simulink model "nona_13_12_simscape_4QC_real"  (R2021b)
settings: Solver=VariableStepAuto  StartTime=0.0  StopTime=10.0  MaxStep=1e-5  RelTol=1e-3
values from neighbouring files (symbols this model uses):
  fsw = 10000    [simul_parameters.m]
  kt = 16.7*10^(-3)    (= 0.0167)    [simul_parameters.m]
libraries: nesl_utility x12, ee_lib x11, fl_lib x8, simulink x1
settings Model: Creator=claudio.rossi  LastModifiedBy=karim

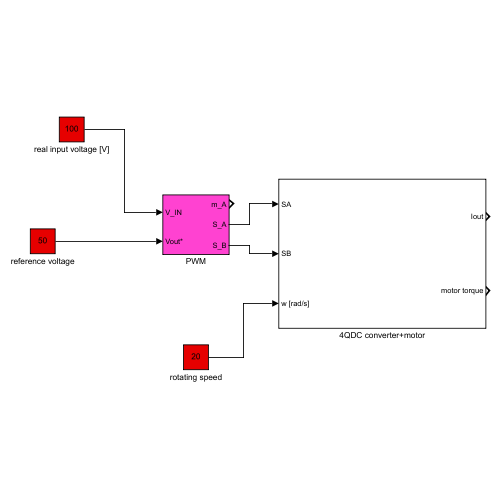
[thumbnail: Simulink's stored preview of the top-level diagram]
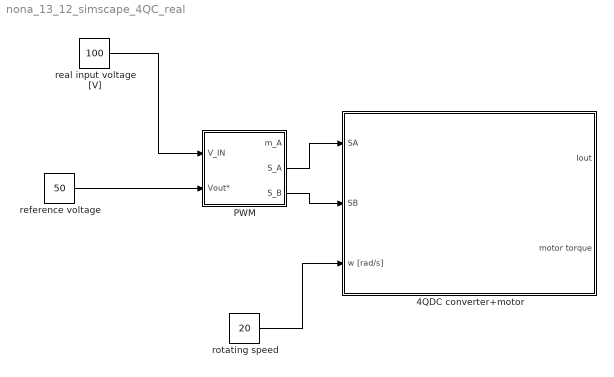
== system nona_13_12_simscape_4QC_real ==
  4QDC converter+motor : Subsystem
  PWM : Subsystem
  real input voltage [V] : Constant  Value=100
  reference voltage : Constant  Value=50
  rotating speed : Constant  Value=20
  wires:
  PWM/2(S_A) -> 4QDC converter+motor/1(SA)
  PWM/3(S_B) -> 4QDC converter+motor/2(SB)
  real input voltage [V]/1 -> PWM/1(V_IN)
  reference voltage/1 -> PWM/2(Vout*)
  rotating speed/1 -> 4QDC converter+motor/3(w [rad/s])

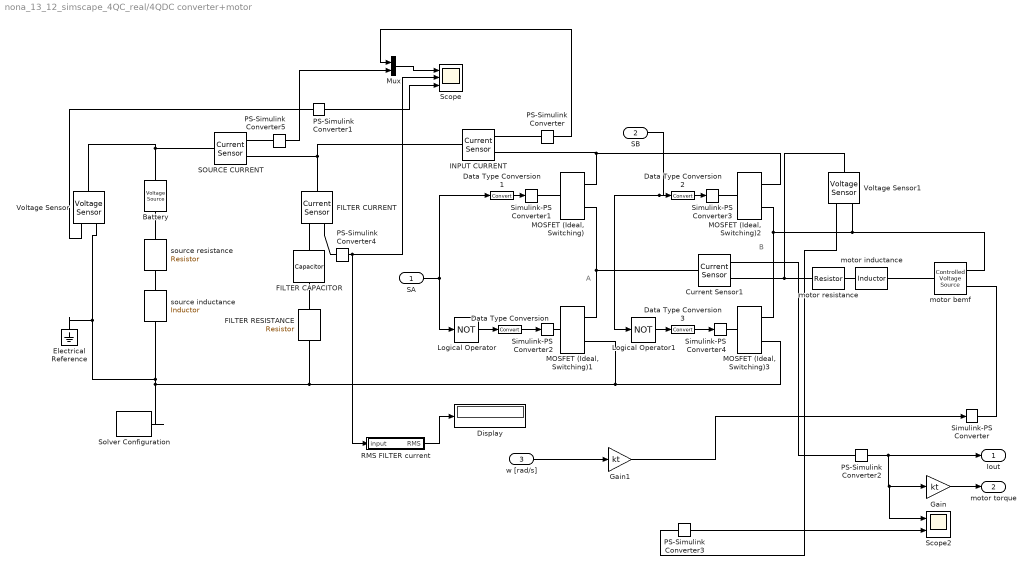
== system nona_13_12_simscape_4QC_real/4QDC converter+motor ==
  note: B
  note: A
  SA : Inport
  SB : Inport  Port=2
  w [rad/s] : Inport  Port=3
  Battery : ee_lib/Sources/Voltage Source  dc_voltage=18 V  ac_voltage=0 V  ac_shift=0 rad  ac_frequency=60 Hz  noise_mode=0  PSD=0 V^2/Hz  repeatability=1  auto_seed=4081172623  user_seed=0  sample_time=1e-3 s  i_specify=off  i_priority=None  i=0 A  i_nominal_specify=off  i_nominal_unit=A  i_nominal_value=1  v_specify=off  v_priority=None  v=0 V  v_nominal_specify=off  v_nominal_unit=V  v_nominal_value=1
  Current Sensor1 : fl_lib/Electrical/Electrical Sensors/Current Sensor
  Data Type Conversion{,1..3} (4 alike) : DataTypeConversion
  Display : Display
  Electrical Reference : fl_lib/Electrical/Electrical Elements/Electrical Reference
  FILTER CAPACITOR : ee_lib/Passive/Capacitor  cap_option=0  c=940e-6 F  Cvec=[1e-05, 1e-06] F  Vvec=[0, 10] V  CV_table_symmetry=1  f_vec=[1, 10] kHz  DFext_vec=[.8, 1.2]  C_tol=5  enable_C_tol=0  tol_distribution=1  nSigma=4  r=0.21 Ohm  g=0 1/Ohm  averaging_period=0 s  enable_operating_limits=0  operating_limit_action=2  max_working_voltage_range=[-25, 25] V  power_rating=1 W  enable_faults=0  fault_action=1  Cscale_faulted=100  R_faulted=1e-3 Ohm  G_faulted=0 1/Ohm  tau_fault=1e-3 s  enable_temporal_fault=0  t_fault=1 s  enable_behavioral_fault=0  max_permissible_voltage_range=[-100, 100] V  t_fail_on_voltage=1 s  i_specify=off  i_priority=None  i=0 A  i_nominal_specify=off  i_nominal_unit=A  i_nominal_value=1  v_specify=off  v_priority=None  v=0 V  v_nominal_specify=off  v_nominal_unit=V  v_nominal_value=1  vc_specify=off  vc_priority=High  vc=0 V  vc_nominal_specify=off  vc_nominal_unit=V  vc_nominal_value=1
  FILTER CURRENT : fl_lib/Electrical/Electrical Sensors/Current Sensor
  FILTER RESISTANCE : ee_lib/Passive/Resistor  R=2 Ohm  R_tol=5  enable_R_tol=0  tol_distribution=1  nSigma=4  enable_operating_limits=0  operating_limit_action=2  max_working_voltage=100 V  power_rating=1 W  enable_faults=0  fault_action=1  R_faulted=inf Ohm  enable_temporal_fault=0  t_fault=1 s  enable_behavioral_fault=0  max_permissible_current=1 A  t_fail_on_current=1 s  noise_mode=0  sample_time=1e-3 s  repeatability=1  auto_seed=2350272805  user_seed=0  Tdevice=25 degC  power_derating_T1=70 degC  power_derating_T2=155 degC  operating_temperature_range_vec=[-50, 150] degC  alpha=3.93e-3 1/K  Tmeas=25 degC  thermal_mass=100 J/K  temperature_specify=off  temperature_priority=High  temperature=298.15 K  temperature_nominal_specify=off  temperature_nominal_unit=K  temperature_nominal_value=1
  Gain : Gain  Gain=kt
  Gain1 : Gain  Gain=kt
  INPUT CURRENT : fl_lib/Electrical/Electrical Sensors/Current Sensor
  Logical Operator : Logic  Operator=NOT  AllPortsSameDT=off  OutDataTypeStr=boolean
  Logical Operator1 : Logic  Operator=NOT  AllPortsSameDT=off  OutDataTypeStr=boolean
  MOSFET (Ideal, Switching){,1..3} (4 alike) : ee_lib/Semiconductors & Converters/MOSFET (Ideal, Switching)  Rds=0.01 Ohm  Goff=1e-6 1/Ohm  Vth=0.5 V  diode_param=1  diode_Vf=0.8 V  diode_Ron=0.001 Ohm  diode_Goff=1e-5 1/Ohm  diode_C=50e-9 F  diode_iRM=-235 A  diode_iF=300 A  diode_idot=-50 A/us  diode_trr_param=1  diode_trr_factor=3  diode_trr=15 us  diode_Qrr=1500 s*uA  thermal_loss_option=ee.enum.converters.thermalLossOption.constantvalues  Von_data=[0, 1.1, 1.3, 1.45, 1.75, 2.25, 2.7; 0, 1, 1.15, 1.35, 1.7, 2.35, 3] V  Tj=[298.15, 398.15] K  Iout_data=[0, 10, 50, 100, 200, 400, 600] A  Eon_data=[0, .29, 1.43, 2.86, 5.71, 13.14, 22.86; 0, .57, 2.63, 5.14, 10.29, 20.57, 30.29] * 1e-3 J  Eoff_data=[0, .21, 1.07, 2.14, 4.29, 9.86, 17.14; 0, .43, 1.97, 3.86, 7.71, 15.43, 22.71] * 1e-3 J  Tj_loss=[298.15, 398.15] K  Iout_data_loss=[0, 10, 50, 100, 200, 400, 600] A  Eon_scalar=22.86e-3 J  Eoff_scalar=17.14e-3 J  Voff=300 V  Iout_scalar=600 A  diodeModelType=ee.enum.converters.diodeModelType.pwl  diodeTableType=ee.enum.diode.tableType.IfMat  diode_IfMat=[.07, .12, .19, 1.75, 4.24, 7.32, 11.2; .16, .3, .72, 2.14, 4.02, 6.35, 9.12] A  diode_VfMat=[.9, 1.15, 1.25, 1.5, 1.75, 2.17, 2.6, 2.85; .58, .68, .75, 1.1, 1.38, 1.77, 2.27, 2.7] V  diode_TjVec=[25, 125] degC  diode_VfVec=[.5, .7, .9, 1.3, 1.7, 2.1, 2.5] V  diode_IfVec=[.1, .2, .5, 1, 2, 4, 7, 10] A  diode_Vr=-600 V  diode_Ls=150 nH  diode_Erec=0.03 J  thermal_network_parameterization=ee.enum.thermalNetworkTopology.external  Rth=[.03, .2] K/W  Rth_Cauer=[.03, .1, .2] K/W  Rth_Foster=[.03, .2] K/W  thermal_mass_parameterization=ee.enum.thermalNetwork.timeconstant  thermal_mass=[3, 25] J/K  thermal_mass_Cauer=[3, 10, 25] J/K  thermal_mass_Foster=[33, 50] J/K  thermal_time_constant=[.1, 5] s  thermal_time_constant_Cauer=[.1, 1, 5] s  thermal_time_constant_Foster=[1, 10] s  thermal_mass_initial_temperatures=[25, 25] degC  thermal_mass_initial_temperatures_Cauer=[25, 25, 25] degC  junction_thermal_mass=0.1 J/K  steadyState_Foster=simscape.enum.onoff.on  Tvec_initial_Foster=[25, 25, 25, 25] degC  no_thermal_network=0  junction_temperature_specify=off  junction_temperature_priority=None  junction_temperature=25 degC  junction_temperature_nominal_specify=off  junction_temperature_nominal_unit=degC  junction_temperature_nominal_value=1  vT_specify=off  vT_priority=None  vT=0 V  vT_nominal_specify=off  vT_nominal_unit=V  vT_nominal_value=1  Qj_specify=off  Qj_priority=None  Qj=0 W  Qj_nominal_specify=off  Qj_nominal_unit=W  Qj_nominal_value=1
  Mux : Mux  Inputs=2
  PS-Simulink Converter{,1..5} (6 alike) : nesl_utility/PS-Simulink Converter  PhysicalDomain=network_engine_domain  SubClassName=ps_output  LeftPortType=input  RightPortType=output  PseudoPeriodic=off  Frequencies=[]  Unit=inherit  AffineConversion=off
      settings: SourceProductBaseCode=PW,SS
  RMS FILTER current : Subsystem  mask{t=1/fsw}
      mask prompts: t "Integrating time T [s]"
      mask DialogControl DescTextVar Prompt: Mean value calculator over period T
  SOURCE CURRENT : fl_lib/Electrical/Electrical Sensors/Current Sensor
  Scope : Scope  NumInputPorts=3
  Scope2 : Scope  NumInputPorts=2
  Simulink-PS Converter{,1..4} (5 alike) : nesl_utility/Simulink-PS Converter  PhysicalDomain=network_engine_domain  SubClassName=ps_input  LeftPortType=input  RightPortType=output  PseudoPeriodic=off  Frequencies=[]  NoiseDistribution=none  NoiseParameters=[]  Unit=1  AffineConversion=off  FilteringAndDerivatives=provide  SimscapeFilterOrder=1  InputFilterTimeConstant=0.001  UdotUserProvided=0
      settings: SourceProductBaseCode=PW,SS
  Solver Configuration : nesl_utility/Solver Configuration  PhysicalDomain=network_engine_domain  SubClassName=solver  LeftPortType=input  RightPortType=generic  Tones=[]  Harmonics=[]  SimulateNoise=off  Profile=off  UseLocalSampling=off  EnableSwitchedLinearOptims=on  FrequencyDomain=off  UseCCode=off  RelTol=0.001  AbsTol=1e-06  MinStep=1e-09  ToWorkspace=off  RevertToSquareIcSolve=off  NumHomotopyIterations=100  PhasorMode=off  PhasorModeNumHarmonics=1  DoDC=off  ResidualTolerance=1e-09  UseLocalSolver=off  LocalSolverChoice=NE_BACKWARD_EULER_ADVANCER  LocalSolverSampleTime=0.001  DoFixedCost=off  MaxNonlinIter=3  MaxModeIter=2  ComputeImpulses=off  ImpulseIterations=2  LinearAlgebra=auto  EquationFormulation=NE_TIME_EF  DelaysMemoryBudget=1024  AutomaticFiltering=on  FilteringTimeConstant=0.001  PartitionStorageMethod=AS_NEEDED  PartitionMemoryBudget=1024  PartitionMethod=ROBUST
      settings: SourceProductBaseCode=PW,SS
  Voltage Sensor : fl_lib/Electrical/Electrical Sensors/Voltage Sensor
  Voltage Sensor1 : fl_lib/Electrical/Electrical Sensors/Voltage Sensor
  motor inductance : ee_lib/Passive/Inductor  l=0.0245 mH  L_tol=20  enable_L_tol=0  tol_distribution=1  nSigma=4  r=0 Ohm  g=1e-9 1/Ohm  enable_operating_limits=0  operating_limit_action=2  max_working_current=1 A  power_rating=1 W  enable_faults=0  fault_action=1  lambdaPercent=50  k_faulted=0.9999  turnsShort=0  openCct=0  groundShort=0  groundShortG=0 1/Ohm  tau_fault=1e-3 s  enable_temporal_fault=0  t_fault=1 s  enable_behavioral_fault=0  max_permissible_voltage=100 V  n_fail_on_voltage=1  max_permissible_current=1 A  t_fail_on_current=1 s  i_L_specify=off  i_L_priority=High  i_L=0 A  i_L_nominal_specify=off  i_L_nominal_unit=A  i_L_nominal_value=1
  "motor resistance " : ee_lib/Passive/Resistor  R=0.12 Ohm  R_tol=5  enable_R_tol=0  tol_distribution=1  nSigma=4  enable_operating_limits=0  operating_limit_action=2  max_working_voltage=100 V  power_rating=1 W  enable_faults=0  fault_action=1  R_faulted=inf Ohm  enable_temporal_fault=0  t_fault=1 s  enable_behavioral_fault=0  max_permissible_current=1 A  t_fail_on_current=1 s  noise_mode=0  sample_time=1e-3 s  repeatability=1  auto_seed=147944790  user_seed=0  Tdevice=25 degC  power_derating_T1=70 degC  power_derating_T2=155 degC  operating_temperature_range_vec=[-50, 150] degC  alpha=3.93e-3 1/K  Tmeas=25 degC  thermal_mass=100 J/K  temperature_specify=off  temperature_priority=High  temperature=298.15 K  temperature_nominal_specify=off  temperature_nominal_unit=K  temperature_nominal_value=1
  motor bemf : fl_lib/Electrical/Electrical Sources/Controlled Voltage Source
  source inductance : ee_lib/Passive/Inductor  l=0.72 mH  L_tol=20  enable_L_tol=0  tol_distribution=1  nSigma=4  r=0 Ohm  g=1e-9 1/Ohm  enable_operating_limits=0  operating_limit_action=2  max_working_current=1 A  power_rating=1 W  enable_faults=0  fault_action=1  lambdaPercent=50  k_faulted=0.9999  turnsShort=0  openCct=0  groundShort=0  groundShortG=0 1/Ohm  tau_fault=1e-3 s  enable_temporal_fault=0  t_fault=1 s  enable_behavioral_fault=0  max_permissible_voltage=100 V  n_fail_on_voltage=1  max_permissible_current=1 A  t_fail_on_current=1 s  i_L_specify=off  i_L_priority=High  i_L=0 A  i_L_nominal_specify=off  i_L_nominal_unit=A  i_L_nominal_value=1
  source resistance : ee_lib/Passive/Resistor  R=0.72 Ohm  R_tol=5  enable_R_tol=0  tol_distribution=1  nSigma=4  enable_operating_limits=0  operating_limit_action=2  max_working_voltage=100 V  power_rating=1 W  enable_faults=0  fault_action=1  R_faulted=inf Ohm  enable_temporal_fault=0  t_fault=1 s  enable_behavioral_fault=0  max_permissible_current=1 A  t_fail_on_current=1 s  noise_mode=0  sample_time=1e-3 s  repeatability=1  auto_seed=471852434  user_seed=0  Tdevice=25 degC  power_derating_T1=70 degC  power_derating_T2=155 degC  operating_temperature_range_vec=[-50, 150] degC  alpha=3.93e-3 1/K  Tmeas=25 degC  thermal_mass=100 J/K  temperature_specify=off  temperature_priority=High  temperature=298.15 K  temperature_nominal_specify=off  temperature_nominal_unit=K  temperature_nominal_value=1
  Iout : Outport
  motor torque : Outport  Port=2
  wires:
  SB/1 -> Logical Operator1/1, Data Type Conversion2/1
  SA/1 -> Logical Operator/1, Data Type Conversion1/1
  PS-Simulink Converter2/1 -> Scope2/1, Gain/1, Iout/1
  Gain/1 -> motor torque/1
  w [rad/s]/1 -> Gain1/1
  Gain1/1 -> Simulink-PS Converter/1
  PS-Simulink Converter3/1 -> Scope2/2
  Logical Operator/1 -> Data Type Conversion/1
  Data Type Conversion/1 -> Simulink-PS Converter2/1
  Data Type Conversion1/1 -> Simulink-PS Converter1/1
  Data Type Conversion2/1 -> Simulink-PS Converter3/1
  Logical Operator1/1 -> Data Type Conversion3/1
  Data Type Conversion3/1 -> Simulink-PS Converter4/1
  PS-Simulink Converter/1 -> Mux/1
  Mux/1 -> Scope/1
  PS-Simulink Converter1/1 -> Scope/3
  PS-Simulink Converter5/1 -> Mux/2
  PS-Simulink Converter4/1 -> RMS FILTER current/1(input), Scope/2
  RMS FILTER current/1(RMS) -> Display/1
  connections:
  Voltage Sensor/LConn1 -- SOURCE CURRENT/LConn1 -- Battery/LConn1
  "MOSFET (Ideal, Switching)1"/RConn2 -- "MOSFET (Ideal, Switching)3"/RConn2 -- FILTER RESISTANCE/RConn1 -- source inductance/RConn1 -- Electrical Reference/LConn1 -- Voltage Sensor/RConn2 -- Solver Configuration/RConn1
  "motor resistance "/RConn1 -- motor inductance/LConn1
  Simulink-PS Converter3/RConn1 -- "MOSFET (Ideal, Switching)2"/LConn1
  INPUT CURRENT/RConn2 -- "MOSFET (Ideal, Switching)2"/RConn1 -- "MOSFET (Ideal, Switching)"/RConn1
  "MOSFET (Ideal, Switching)3"/RConn1 -- motor bemf/RConn2 -- Voltage Sensor1/RConn2 -- "MOSFET (Ideal, Switching)2"/RConn2
  INPUT CURRENT/RConn1 -- PS-Simulink Converter/LConn1
  Voltage Sensor/RConn1 -- PS-Simulink Converter1/LConn1
  Simulink-PS Converter1/RConn1 -- "MOSFET (Ideal, Switching)"/LConn1
  Simulink-PS Converter/RConn1 -- motor bemf/RConn1
  "MOSFET (Ideal, Switching)"/RConn2 -- "MOSFET (Ideal, Switching)1"/RConn1 -- Current Sensor1/LConn1
  Simulink-PS Converter4/RConn1 -- "MOSFET (Ideal, Switching)3"/LConn1
  Simulink-PS Converter2/RConn1 -- "MOSFET (Ideal, Switching)1"/LConn1
  motor inductance/RConn1 -- motor bemf/LConn1
  Current Sensor1/RConn2 -- Voltage Sensor1/LConn1 -- "motor resistance "/LConn1
  Current Sensor1/RConn1 -- PS-Simulink Converter2/LConn1
  Voltage Sensor1/RConn1 -- PS-Simulink Converter3/LConn1
  source inductance/LConn1 -- source resistance/RConn1
  source resistance/LConn1 -- Battery/RConn1
  SOURCE CURRENT/RConn2 -- FILTER CURRENT/LConn1 -- INPUT CURRENT/LConn1
  FILTER CURRENT/RConn2 -- FILTER CAPACITOR/LConn1
  FILTER CURRENT/RConn1 -- PS-Simulink Converter4/LConn1
  SOURCE CURRENT/RConn1 -- PS-Simulink Converter5/LConn1
  FILTER CAPACITOR/RConn1 -- FILTER RESISTANCE/LConn1

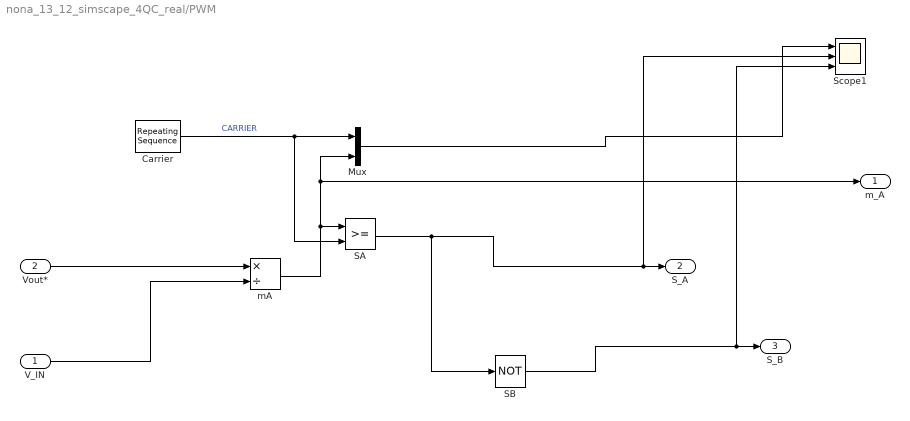
== system nona_13_12_simscape_4QC_real/PWM ==
  V_IN : Inport
  Vout* : Inport  Port=2
  Carrier : simulink/Sources/Repeating Sequence  rep_seq_t="[0 1/fsw/2  1/fsw]"  rep_seq_y=[-1 1 -1]
  Mux : Mux  Inputs=2
  SA : RelationalOperator  OutDataTypeStr=boolean  RndMeth=Simplest
  SB : Logic  Operator=NOT  AllPortsSameDT=off  OutDataTypeStr=boolean
  Scope1 : Scope  NumInputPorts=3
  mA : Product  Inputs=*/
  m_A : Outport
  S_A : Outport  Port=2
  S_B : Outport  Port=3
  wires:
  Carrier/1 -> SA/2, Mux/1  "CARRIER"
  V_IN/1 -> mA/2
  SA/1 -> SB/1, Scope1/2, S_A/1
  Mux/1 -> Scope1/1
  Vout*/1 -> mA/1
  mA/1 -> Mux/2, m_A/1, SA/1
  SB/1 -> Scope1/3, S_B/1

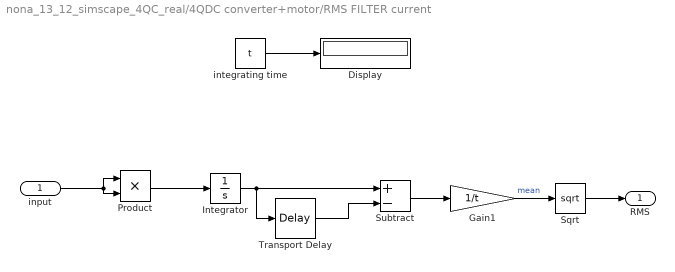
== system nona_13_12_simscape_4QC_real/4QDC converter+motor/RMS FILTER current ==
  input : Inport
  Display : Display
  Gain1 : Gain  Gain=1/t
  Integrator : Integrator
  Product : Product
  Sqrt : Sqrt  SaturateOnIntegerOverflow=on
  Subtract : Sum  Inputs=+-
  Transport Delay : TransportDelay  DelayTime=t
  integrating time : Constant  Value=t
  RMS : Outport
  wires:
  integrating time/1 -> Display/1
  Transport Delay/1 -> Subtract/2
  Integrator/1 -> Transport Delay/1, Subtract/1
  Subtract/1 -> Gain1/1
  input/1 -> Product/1, Product/2
  Product/1 -> Integrator/1
  Sqrt/1 -> RMS/1
  Gain1/1 -> Sqrt/1  "mean"
